simulink model "SOC_codegen"  (R2024b)
settings: Solver=ode4  StartTime=0.0  StopTime=10.0  FixedStep=0.01  RelTol=1e-3  EnableMultiTasking=on
undefined symbols (not defined in the file): C_OcvTable, C_SocTable, DiscIntNeverNeededParam, SOCc_CapacityFilterCoeff, SOCk_CellBalancingResistor, SOCk_CellCapacity, SOCk_HrsToSec, SOCk_NumberInSeries, SOCk_SocMaxPercentage, SOCk_SocMinPercentage, SOCk_stepSize, SOCk_ToFractionFromPercentage, SOCk_ToPercentage, SOCv_factoryInitSohC, SOCv_InitalSOC
libraries: simulink x2
settings Model: Creator=nctzv8  LastModifiedBy=voillat
settings SolverCC: AlgebraicLoopSolver=TrustRegion
settings DataIOCC: LimitDataPoints=on  SignalLogging=off  DSMLogging=off
settings OptimizationCC: DefaultParameterBehavior=Inlined  EnhancedBackFolding=on  PassReuseOutputArgsAs=Individual arguments  ZeroExternalMemoryAtStartup=off  ZeroInternalMemoryAtStartup=off  OptimizeBlockOrder=speed  DifferentSizesBufferReuse=on  OptimizationCustomize=off  EfficientTunableParamExpr=on
settings DebuggingCC: ParameterTunabilityLossMsg=error  UnconnectedInputMsg=warning  UnconnectedOutputMsg=warning  UnconnectedLineMsg=warning  AllowSymbolicDim=off  SFUnexpectedBacktrackingDiag=warning  SFNoUnconditionalDefaultTransitionDiag=warning  SFExecutionAtInitializationDiag=none  ArithmeticOperatorsInVariantConditions=warning
settings ModelReferenceCC: EnableRefExpFcnMdlSchedulingChecks=on  PropagateSignalLabelsOutOfModel=off
settings SFSimCC: SimUseLocalCustomCode=off  MATLABDynamicMemAlloc=off  CustomCodeUndefinedFunction=UseInterfaceOnly
settings RTWCC: Description=Embedded Coder  SystemTargetFile=ert.tlc  GenCodeOnly=on  TemplateMakefile=ert_default_tmf  GenerateReport=on  RTWUseLocalCustomCode=off  GPUComputeCapability=3.5  DLArmComputeVersion=19.05
settings CodeAppCC: ForceParamTrailComments=on  IgnoreCustomStorageClasses=off  OperatorAnnotations=on  SimulinkDataObjDesc=on  SFDataObjDesc=on  InsertBlockDesc=on  ReqsInCode=on
settings ERTTargetCC: GenerateSampleERTMain=on  ERTCustomFileTemplate=example_file_process.tlc  DynamicArrayContainerType=coder::array
settings ConfigComp: CovMetricSettings=dw  CovSaveCumulativeToWorkspaceVar=on  CovSaveSingleToWorkspaceVar=on  CovExternalEMLEnable=off

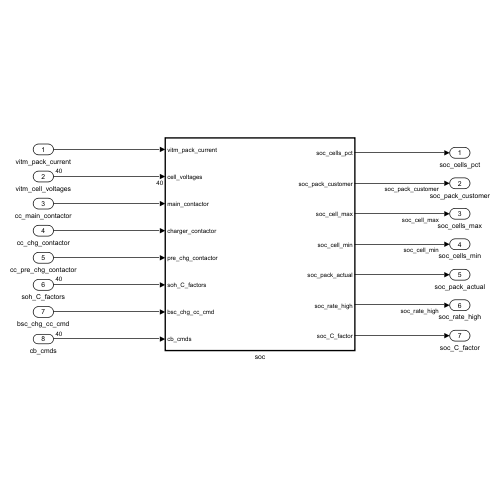
[thumbnail: Simulink's stored preview of the top-level diagram]
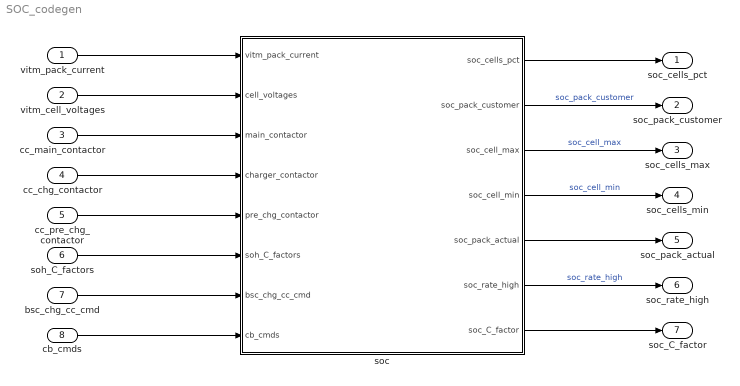
== system SOC_codegen ==
  vitm_pack_current : Inport
  vitm_cell_voltages : Inport  Port=2  PortDimensions=40
  cc_main_contactor : Inport  Port=3
  cc_chg_contactor : Inport  Port=4
  cc_pre_chg_contactor : Inport  Port=5
  soh_C_factors : Inport  Port=6  PortDimensions=40
  bsc_chg_cc_cmd : Inport  Port=7
  cb_cmds : Inport  Port=8  OutDataTypeStr=boolean  PortDimensions=40
  soc : Subsystem  TreatAsAtomicUnit=on
  soc_cells_pct : Outport
  soc_pack_customer : Outport  Port=2
  soc_cells_max : Outport  Port=3
  soc_cells_min : Outport  Port=4
  soc_pack_actual : Outport  Port=5
  soc_rate_high : Outport  Port=6
  soc_C_factor : Outport  Port=7  InitialOutput=ones(40,1)
  wires:
  vitm_pack_current/1 -> soc/1(vitm_pack_current)
  vitm_cell_voltages/1 -> soc/2(cell_voltages)
  cc_main_contactor/1 -> soc/3(main_contactor)
  cc_pre_chg_contactor/1 -> soc/5(pre_chg_contactor)
  soc/1(soc_cells_pct) -> soc_cells_pct/1
  soc/2(soc_pack_customer) -> soc_pack_customer/1  "soc_pack_customer"
  soc/3(soc_cell_max) -> soc_cells_max/1  "soc_cell_max"
  soc/4(soc_cell_min) -> soc_cells_min/1  "soc_cell_min"
  soc/5(soc_pack_actual) -> soc_pack_actual/1
  soc/6(soc_rate_high) -> soc_rate_high/1  "soc_rate_high"
  cc_chg_contactor/1 -> soc/4(charger_contactor)
  soh_C_factors/1 -> soc/6(soh_C_factors)
  soc/7(soc_C_factor) -> soc_C_factor/1
  bsc_chg_cc_cmd/1 -> soc/7(bsc_chg_cc_cmd)
  cb_cmds/1 -> soc/8(cb_cmds)

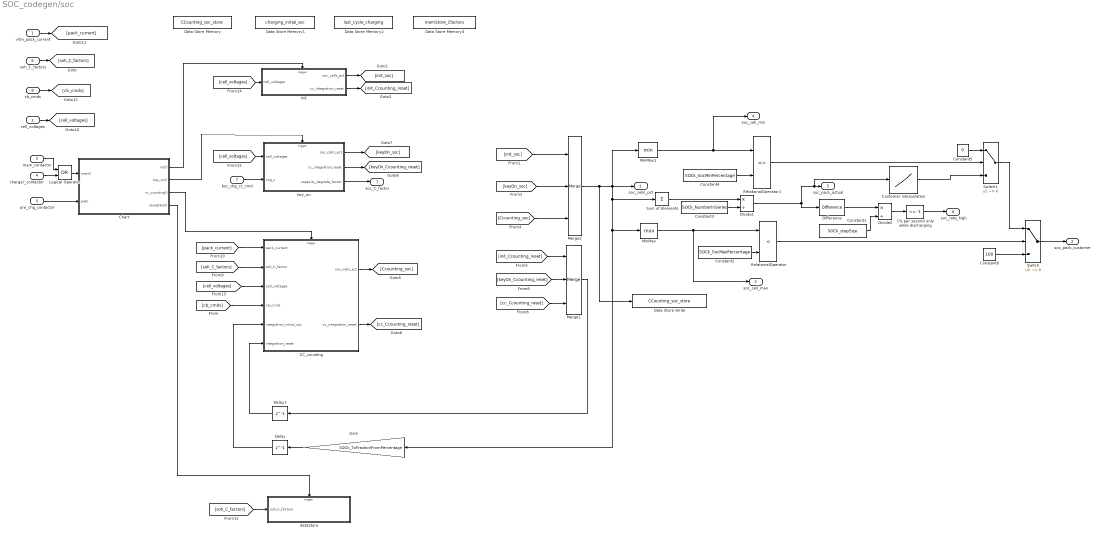
== system SOC_codegen/soc ==
  vitm_pack_current : Inport
  cell_voltages : Inport  Port=2  PortDimensions=40
  main_contactor : Inport  Port=3
  charger_contactor : Inport  Port=4
  pre_chg_contactor : Inport  Port=5
  soh_C_factors : Inport  Port=6
  bsc_chg_cc_cmd : Inport  Port=7
  cb_cmds : Inport  Port=8
  1% per second only while discharging : simulink/Logic and Bit Operations/Compare To Constant  relop=<=  const=-1  OutDataTypeStr=boolean
  CC_counting : Subsystem
  Chart : Stateflow chart  TreatAsAtomicUnit=on
  Constant1 : Constant  Value=SOCk_stepSize  SampleTime=-1
  Constant2 : Constant  Value=SOCk_SocMaxPercentage
  Constant3 : Constant  Value=SOCk_NumberInSeries
  Constant4 : Constant  Value=SOCk_SocMinPercentage
  Constant5 : Constant  Value=0
  Constant6 : Constant  Value=100
  Customer interpolation : Lookup_n-D  NumberOfTableDimensions=1  BreakpointsForDimension1=[SOCk_SocMinPercentage SOCk_SocMaxPercentage]  Table=[0 100]  InternalRulePriority=Speed  RndMeth=Simplest
  Data Store Memory : DataStoreMemory  DataStoreName=CCounting_soc_store  ReadBeforeWriteMsg=warning  WriteAfterWriteMsg=warning  WriteAfterReadMsg=warning  InitialValue=SOCv_InitalSOC  ShowAdditionalParam=off
  Data Store Memory1 : DataStoreMemory  DataStoreName=charging_initial_soc  ReadBeforeWriteMsg=warning  WriteAfterWriteMsg=warning  WriteAfterReadMsg=warning  InitialValue=SOCv_InitalSOC  ShowAdditionalParam=off
  Data Store Memory2 : DataStoreMemory  DataStoreName=last_cycle_charging  ReadBeforeWriteMsg=warning  WriteAfterWriteMsg=warning  WriteAfterReadMsg=warning  ShowAdditionalParam=off
  Data Store Memory3 : DataStoreMemory  DataStoreName=memStore_Cfactors  ReadBeforeWriteMsg=warning  WriteAfterWriteMsg=warning  WriteAfterReadMsg=warning  InitialValue=SOCv_factoryInitSohC  ShowAdditionalParam=off
  Data Store Write : DataStoreWrite  DataStoreName=CCounting_soc_store  IndexOptions=Index vector (dialog)  Indices=1  OutputSizes=1
  Delay : Delay  DelayLength=1  InitialCondition=SOCv_InitalSOC
  Delay1 : Delay  DelayLength=1  InitialCondition=0
  Difference : simulink/Discrete/Difference  ICPrevInput=0.0  OutMin=[]  OutMax=[]  OutDataType=fixdt(1, 16)  OutScaling=2^-10  DoSatur=off
  Divide1 : Product  Inputs=*/
  Divide2 : Product  Inputs=*/
  Gain : Gain  Gain=SOCk_ToFractionFromPercentage
  Init : Subsystem
  Logical Operator : Logic  Operator=OR  AllPortsSameDT=off  OutDataTypeStr=boolean
  Merge1 : Merge  Inputs=3
  Merge2 : Merge  Inputs=3
  MinMax : MinMax  Function=max
  MinMax1 : MinMax
  RelationalOperator : RelationalOperator  Operator=<  OutDataTypeStr=boolean  InputSameDT=off
  RelationalOperator1 : RelationalOperator  Operator=<=  OutDataTypeStr=boolean  InputSameDT=off
  Sum of Elements : Sum  Inputs=+
  Switch : Switch  Criteria=u2 ~= 0  SaturateOnIntegerOverflow=off  InputSameDT=off
  Switch1 : Switch  Criteria=u2 ~= 0  SaturateOnIntegerOverflow=off  InputSameDT=off
  dataStore : Subsystem
  key_on : Subsystem
  soc_cells_pct : Outport
  soc_pack_customer : Outport  Port=2
  soc_cell_max : Outport  Port=3
  soc_cell_min : Outport  Port=4
  soc_pack_actual : Outport  Port=5
  soc_rate_high : Outport  Port=6
  soc_C_factor : Outport  Port=7
  wires:
  Switch/1 -> soc_pack_customer/1
  Customer interpolation/1 -> Switch1/3
  Constant1/1 -> Divide2/2
  Difference/1 -> Divide2/1
  Divide2/1 -> 1% per second only while discharging/1
  key_on/3(capacity_degrade_factor) -> soc_C_factor/1
  [cell_voltages] -> key_on/1(cell_voltages)
  [cell_voltages] -> Init/1(cell_voltages)
  cell_voltages/1 -> [cell_voltages]
  [cell_voltages] -> CC_counting/3(cell_voltages)
  [cb_cmds] -> CC_counting/4(cb_cmds)
  cb_cmds/1 -> [cb_cmds]
  [soh_C_factors] -> dataStore/1(soh_C_factors)
  Chart/4(saveData()) -> dataStore/Trigger
  [pack_current] -> CC_counting/1(pack_current)
  bsc_chg_cc_cmd/1 -> key_on/2(chg_c)
  soh_C_factors/1 -> [soh_C_factors]
  [soh_C_factors] -> CC_counting/2("soh_C_factor ")
  [cc_Ccounting_reset] -> Merge1/3
  [keyOn_Ccounting_reset] -> Merge1/2
  [init_Ccounting_reset] -> Merge1/1
  [Ccounting_soc] -> Merge2/3
  [keyOn_soc] -> Merge2/2
  [init_soc] -> Merge2/1
  key_on/2(cc_integration_reset) -> [keyOn_Ccounting_reset]
  key_on/1(soc_cells_pct) -> [keyOn_soc]
  CC_counting/2(cc_integration_reset) -> [cc_Ccounting_reset]
  CC_counting/1(soc_cells_pct) -> [Ccounting_soc]
  Init/2(cc_integration_reset) -> [init_Ccounting_reset]
  Init/1(soc_cells_pct) -> [init_soc]
  charger_contactor/1 -> Logical Operator/2
  main_contactor/1 -> Logical Operator/1
  Logical Operator/1 -> Chart/1(mainC)
  Delay1/1 -> CC_counting/6(integration_reset)
  Merge1/1 -> Delay1/1
  Gain/1 -> Delay/1
  Delay/1 -> CC_counting/5(integration_initial_soc)
  Chart/2(key_on()) -> key_on/Trigger
  Merge2/1 -> MinMax1/1, Sum of Elements/1, MinMax/1, Gain/1, soc_cells_pct/1, Data Store Write/1
  1% per second only while discharging/1 -> soc_rate_high/1
  pre_chg_contactor/1 -> Chart/2(preC)
  Chart/1(init()) -> Init/Trigger
  vitm_pack_current/1 -> [pack_current]
  Sum of Elements/1 -> Divide1/1
  Constant4/1 -> RelationalOperator1/2
  RelationalOperator/1 -> Switch/2
  Divide1/1 -> soc_pack_actual/1, Customer interpolation/1, Difference/1
  MinMax/1 -> RelationalOperator/1, soc_cell_max/1
  RelationalOperator1/1 -> Switch1/2
  Switch1/1 -> Switch/1
  Chart/3(cc_counting()) -> CC_counting/Trigger
  Constant2/1 -> RelationalOperator/2
  Constant6/1 -> Switch/3
  Constant5/1 -> Switch1/1
  MinMax1/1 -> RelationalOperator1/1, soc_cell_min/1
  Constant3/1 -> Divide1/2

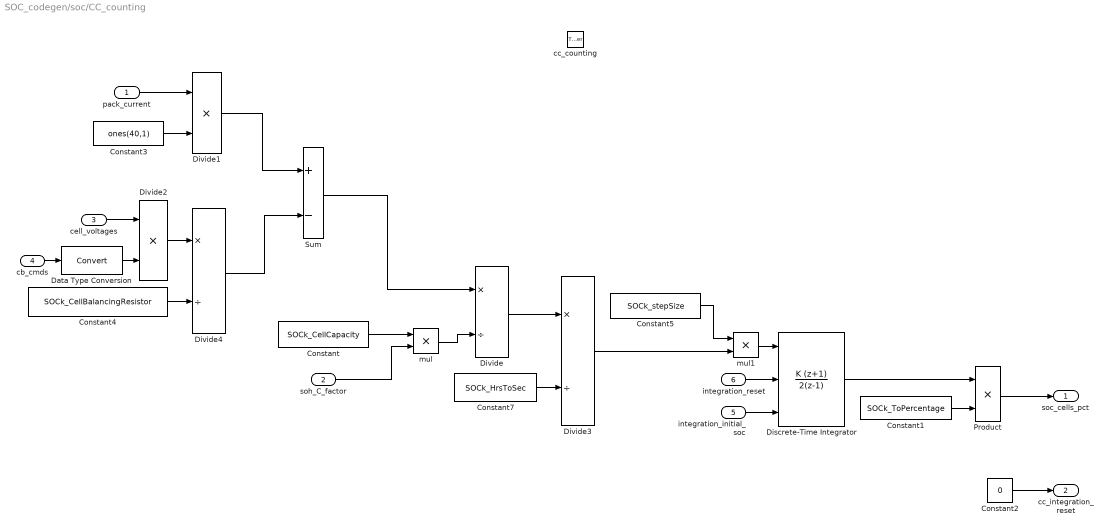
== system SOC_codegen/soc/CC_counting ==
  pack_current : Inport
  "soh_C_factor " : Inport  Port=2
  cell_voltages : Inport  Port=3
  cb_cmds : Inport  Port=4
  integration_initial_soc : Inport  Port=5
  integration_reset : Inport  Port=6
  cc_counting : TriggerPort  TriggerType=function-call  VariantControl=(inherit)  PortDimensions=1
  Constant : Constant  Value=SOCk_CellCapacity
  Constant1 : Constant  Value=SOCk_ToPercentage
  Constant2 : Constant  Value=0
  Constant3 : Constant  Value=ones(40,1)
  Constant4 : Constant  Value=SOCk_CellBalancingResistor
  Constant5 : Constant  Value=SOCk_stepSize  SampleTime=-1
  Constant7 : Constant  Value=SOCk_HrsToSec
  Data Type Conversion : DataTypeConversion  SaturateOnIntegerOverflow=off  RndMeth=Floor
  Discrete-Time Integrator : DiscreteIntegrator  IntegratorMethod=Accumulation: Trapezoidal  ExternalReset=rising  InitialConditionSource=external  SampleTime=-1  LimitOutput=on  ICPrevOutput=DiscIntNeverNeededParam  ICPrevScaledInput=DiscIntNeverNeededParam
  Divide : Product  Inputs=*/
  Divide1 : Product  Inputs=**
  Divide2 : Product  Inputs=**
  Divide3 : Product  Inputs=*/
  Divide4 : Product  Inputs=*/
  Product : Product  RndMeth=Zero
  Sum : Sum  Inputs=+-
  mul : Product  Inputs=**
  mul1 : Product  Inputs=**
  soc_cells_pct : Outport
  cc_integration_reset : Outport  Port=2
  wires:
  Constant5/1 -> mul1/1
  mul1/1 -> Discrete-Time Integrator/1
  Divide3/1 -> mul1/2
  integration_reset/1 -> Discrete-Time Integrator/2
  "soh_C_factor "/1 -> mul/2
  Data Type Conversion/1 -> Divide2/2
  Sum/1 -> Divide/1
  Divide4/1 -> Sum/2
  Divide1/1 -> Sum/1
  Constant4/1 -> Divide4/2
  Divide2/1 -> Divide4/1
  cb_cmds/1 -> Data Type Conversion/1
  cell_voltages/1 -> Divide2/1
  Constant3/1 -> Divide1/2
  pack_current/1 -> Divide1/1
  mul/1 -> Divide/2
  Constant/1 -> mul/1
  Constant2/1 -> cc_integration_reset/1
  Product/1 -> soc_cells_pct/1
  Constant1/1 -> Product/2
  Divide/1 -> Divide3/1
  Constant7/1 -> Divide3/2
  integration_initial_soc/1 -> Discrete-Time Integrator/3
  Discrete-Time Integrator/1 -> Product/1

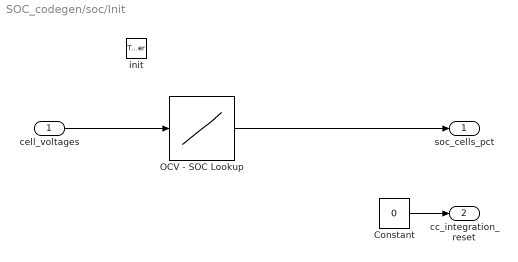
== system SOC_codegen/soc/Init ==
  cell_voltages : Inport
  init : TriggerPort  TriggerType=function-call  VariantControl=(inherit)  PortDimensions=1
  Constant : Constant  Value=0
  OCV - SOC Lookup : Lookup_n-D  NumberOfTableDimensions=1  BreakpointsForDimension1=C_OcvTable  BreakpointsForDimension1FirstPoint=10  BreakpointsForDimension2FirstPoint=10  BreakpointsForDimension1Spacing=12  BreakpointsForDimension2Spacing=12  IndexSearchMethod=Evenly spaced points  Table=C_SocTable  ExtrapMethod=Clip  DiagnosticForOutOfRangeInput=Error  InternalRulePriority=Speed  RndMeth=Simplest
  soc_cells_pct : Outport
  cc_integration_reset : Outport  Port=2
  wires:
  Constant/1 -> cc_integration_reset/1
  OCV - SOC Lookup/1 -> soc_cells_pct/1
  cell_voltages/1 -> OCV - SOC Lookup/1

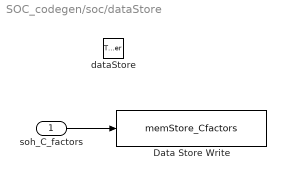
== system SOC_codegen/soc/dataStore ==
  soh_C_factors : Inport
  dataStore : TriggerPort  TriggerType=function-call  VariantControl=(inherit)  PortDimensions=1
  Data Store Write : DataStoreWrite  DataStoreName=memStore_Cfactors  IndexOptions=Index vector (dialog)  Indices=1  OutputSizes=1
  wires:
  soh_C_factors/1 -> Data Store Write/1

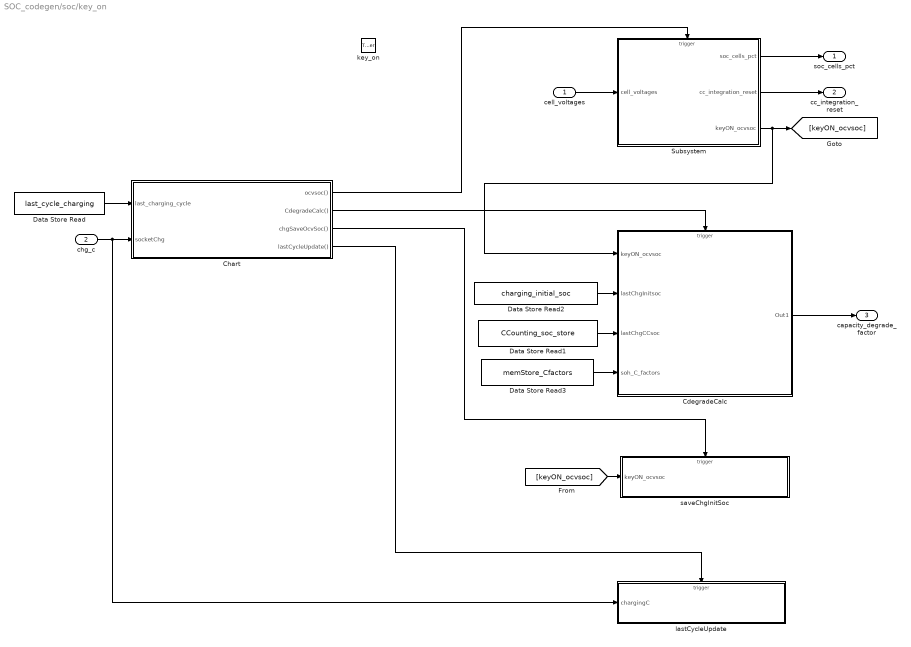
== system SOC_codegen/soc/key_on ==
  cell_voltages : Inport
  chg_c : Inport  Port=2
  key_on : TriggerPort  TriggerType=function-call  VariantControl=(inherit)  PortDimensions=1
  CdegradeCalc : Subsystem
  Chart : Stateflow chart  TreatAsAtomicUnit=on
  Data Store Read : DataStoreRead  DataStoreName=last_cycle_charging  IndexOptions=Index vector (dialog)  Indices=1  OutputSizes=1
  Data Store Read1 : DataStoreRead  DataStoreName=CCounting_soc_store  IndexOptions=Index vector (dialog)  Indices=1  OutputSizes=1
  Data Store Read2 : DataStoreRead  DataStoreName=charging_initial_soc  IndexOptions=Index vector (dialog)  Indices=1  OutputSizes=1
  Data Store Read3 : DataStoreRead  DataStoreName=memStore_Cfactors  IndexOptions=Index vector (dialog)  Indices=1  OutputSizes=1
  Subsystem : Subsystem
  lastCycleUpdate : Subsystem
  saveChgInitSoc : Subsystem
  soc_cells_pct : Outport
  cc_integration_reset : Outport  Port=2
  capacity_degrade_factor : Outport  Port=3  InitialOutput=ones(40,1)
  wires:
  CdegradeCalc/1(Out1) -> capacity_degrade_factor/1
  Chart/2(CdegradeCalc()) -> CdegradeCalc/Trigger
  Chart/3(chgSaveOcvSoc()) -> saveChgInitSoc/Trigger
  Chart/4(lastCycleUpdate()) -> lastCycleUpdate/Trigger
  chg_c/1 -> Chart/2(socketChg), lastCycleUpdate/1(chargingC)
  Chart/1(ocvsoc()) -> Subsystem/Trigger
  Data Store Read3/1 -> CdegradeCalc/4(soh_C_factors)
  Data Store Read/1 -> Chart/1(last_charging_cycle)
  Data Store Read1/1 -> CdegradeCalc/3(lastChgCCsoc)
  Data Store Read2/1 -> CdegradeCalc/2(lastChgInitsoc)
  Subsystem/3(keyON_ocvsoc) -> [keyON_ocvsoc], CdegradeCalc/1(keyON_ocvsoc)
  Subsystem/2(cc_integration_reset) -> cc_integration_reset/1
  Subsystem/1(soc_cells_pct) -> soc_cells_pct/1
  cell_voltages/1 -> Subsystem/1(cell_voltages)
  [keyON_ocvsoc] -> saveChgInitSoc/1(keyON_ocvsoc)

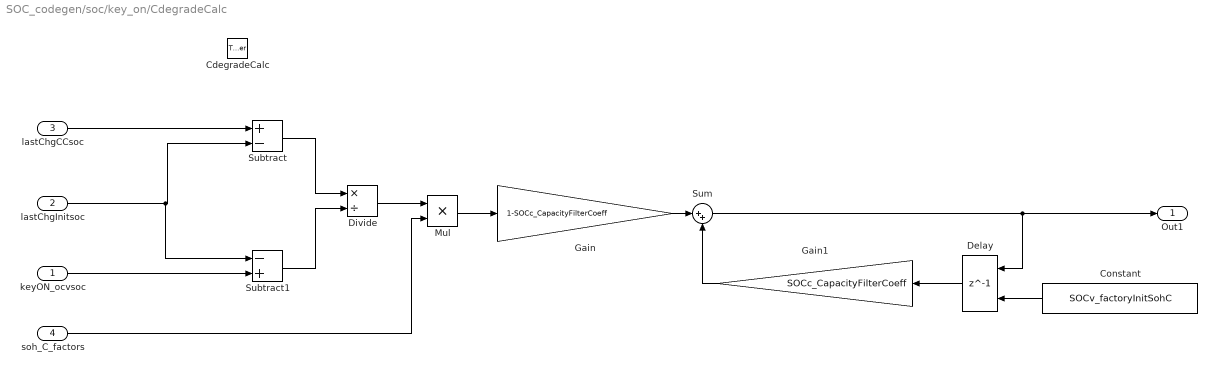
== system SOC_codegen/soc/key_on/CdegradeCalc ==
  keyON_ocvsoc : Inport
  lastChgInitsoc : Inport  Port=2
  lastChgCCsoc : Inport  Port=3
  soh_C_factors : Inport  Port=4
  CdegradeCalc : TriggerPort  TriggerType=function-call  VariantControl=(inherit)  PortDimensions=1
  Constant : Constant  Value=SOCv_factoryInitSohC  SampleTime=-1
  Delay : Delay  DelayLength=1  InitialConditionSource=Input port  InitialCondition=ones(40,1)
      settings: InputPortMap=u0,p4
  Divide : Product  Inputs=*/
  Gain : Gain  Gain=1-SOCc_CapacityFilterCoeff
  Gain1 : Gain  Gain=SOCc_CapacityFilterCoeff
  Mul : Product  Inputs=**
  Subtract : Sum  Inputs=+-
  Subtract1 : Sum  Inputs=-+
  Sum : Sum  Inputs=|++
  Out1 : Outport  InitialOutput=ones(40,1)
  wires:
  Sum/1 -> Out1/1, Delay/1
  keyON_ocvsoc/1 -> Subtract1/2
  Constant/1 -> Delay/2
  Gain1/1 -> Sum/2
  Delay/1 -> Gain1/1
  Gain/1 -> Sum/1
  Mul/1 -> Gain/1
  soh_C_factors/1 -> Mul/2
  lastChgCCsoc/1 -> Subtract/1
  Divide/1 -> Mul/1
  Subtract1/1 -> Divide/2
  Subtract/1 -> Divide/1
  lastChgInitsoc/1 -> Subtract1/1, Subtract/2

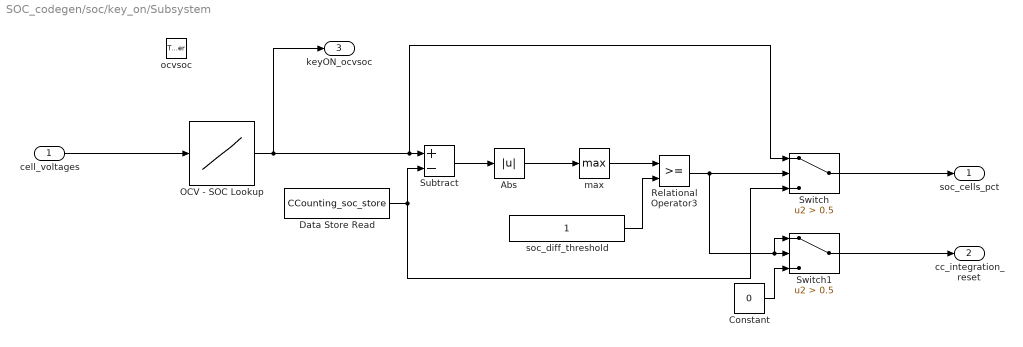
== system SOC_codegen/soc/key_on/Subsystem ==
  cell_voltages : Inport
  ocvsoc : TriggerPort  TriggerType=function-call  VariantControl=(inherit)  PortDimensions=1
  Abs : Abs  SaturateOnIntegerOverflow=off
  Constant : Constant  Value=0
  Data Store Read : DataStoreRead  DataStoreName=CCounting_soc_store  IndexOptions=Index vector (dialog)  Indices=1  OutputSizes=1
  OCV - SOC Lookup : Lookup_n-D  NumberOfTableDimensions=1  BreakpointsForDimension1=C_OcvTable  BreakpointsForDimension1FirstPoint=10  BreakpointsForDimension2FirstPoint=10  BreakpointsForDimension1Spacing=12  BreakpointsForDimension2Spacing=12  IndexSearchMethod=Evenly spaced points  Table=C_SocTable  ExtrapMethod=Clip  DiagnosticForOutOfRangeInput=Error  InternalRulePriority=Speed  RndMeth=Simplest
  Relational Operator3 : RelationalOperator  OutDataTypeStr=boolean  InputSameDT=off
  Subtract : Sum  Inputs=+-
  Switch : Switch  Criteria=u2 > Threshold  Threshold=0.5  SaturateOnIntegerOverflow=off  InputSameDT=off
  Switch1 : Switch  Criteria=u2 > Threshold  Threshold=0.5  SaturateOnIntegerOverflow=off  InputSameDT=off
  max : MinMax  Function=max
  soc_diff_threshold : Constant
  soc_cells_pct : Outport
  cc_integration_reset : Outport  Port=2
  keyON_ocvsoc : Outport  Port=3
  wires:
  cell_voltages/1 -> OCV - SOC Lookup/1
  Relational Operator3/1 -> Switch/2, Switch1/2, Switch1/1
  Constant/1 -> Switch1/3
  OCV - SOC Lookup/1 -> Subtract/1, Switch/1, keyON_ocvsoc/1
  soc_diff_threshold/1 -> Relational Operator3/2
  Switch1/1 -> cc_integration_reset/1
  Subtract/1 -> Abs/1
  Data Store Read/1 -> Subtract/2, Switch/3
  Abs/1 -> max/1
  Switch/1 -> soc_cells_pct/1
  max/1 -> Relational Operator3/1

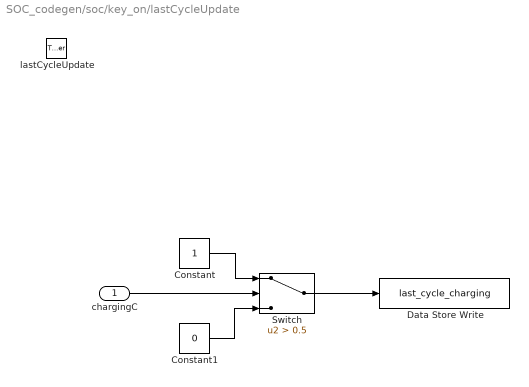
== system SOC_codegen/soc/key_on/lastCycleUpdate ==
  chargingC : Inport
  lastCycleUpdate : TriggerPort  TriggerType=function-call  VariantControl=(inherit)  PortDimensions=1
  Constant : Constant
  Constant1 : Constant  Value=0
  Data Store Write : DataStoreWrite  DataStoreName=last_cycle_charging  IndexOptions=Index vector (dialog)  Indices=1  OutputSizes=1
  Switch : Switch  Criteria=u2 > Threshold  Threshold=0.5  SaturateOnIntegerOverflow=off  InputSameDT=off
  wires:
  Constant1/1 -> Switch/3
  Constant/1 -> Switch/1
  Switch/1 -> Data Store Write/1
  chargingC/1 -> Switch/2

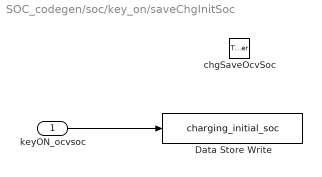
== system SOC_codegen/soc/key_on/saveChgInitSoc ==
  keyON_ocvsoc : Inport
  chgSaveOcvSoc : TriggerPort  TriggerType=function-call  VariantControl=(inherit)  PortDimensions=1
  Data Store Write : DataStoreWrite  DataStoreName=charging_initial_soc  IndexOptions=Index vector (dialog)  Indices=1  OutputSizes=1
  wires:
  keyON_ocvsoc/1 -> Data Store Write/1

== stateflow chart SOC_codegen/soc/Chart ==
  state init
    (default) -> (junction 40)
    init -> (junction 40) [order 1]
    (junction 40) -> (junction 41) : {init;}
  state key_ON
    (default) -> (junction 58)
    key_ON -> (junction 58) [order 1]
    (junction 58) -> (junction 56) : {key_on;}
  state coulomb_counting
    (default) -> (junction 48)
    coulomb_counting -> (junction 48) [order 1]
    (junction 48) -> (junction 46) : {cc_counting;}
  state dataStore
    entry:
    (default) -> (junction 77)
    dataStore -> (junction 77) [order 1]
    (junction 77) -> (junction 74) : {saveData;}
  state end
    entry:
  (default) -> init
  init -> key_ON [order 1] : [preC == 1 || mainC == 1 ]
  end -> key_ON : [preC == 1 || mainC ==1]
  key_ON -> coulomb_counting [order 1] : [preC == 1 || mainC == 1 ]
  coulomb_counting -> dataStore [order 1] : [mainC == 0 && preC == 0]
  dataStore -> end [order 1]
  data: mainC input boolean; preC input boolean
  events: init output FUNCTION_CALL_EVENT; key_on output FUNCTION_CALL_EVENT; cc_counting output FUNCTION_CALL_EVENT; saveData output FUNCTION_CALL_EVENT

== stateflow chart SOC_codegen/soc/key_on/Chart ==
  state keyON
    (default) -> (junction 3)
    keyON -> (junction 3)
    (junction 3) -> (junction 13) : {ocvsoc;}
    (junction 13) -> (junction 14) [order 1] : [last_charging_cycle == 1]
    (junction 13) -> (junction 16) [order 2]
    (junction 14) -> (junction 15) : {CdegradeCalc;}
    (junction 15) -> (junction 16)
    (junction 16) -> (junction 4)
    (junction 4) -> (junction 7) [order 1] : [socketChg == 1]
    (junction 4) -> (junction 6) [order 2]
    (junction 7) -> (junction 10) : {chgSaveOcvSoc;}
    (junction 10) -> (junction 6)
    (junction 6) -> (junction 24) : {lastCycleUpdate;}
  (default) -> keyON
  data: last_charging_cycle input double; socketChg input boolean
  events: ocvsoc output FUNCTION_CALL_EVENT; CdegradeCalc output FUNCTION_CALL_EVENT; chgSaveOcvSoc output FUNCTION_CALL_EVENT; lastCycleUpdate output FUNCTION_CALL_EVENT
